simulink model "TestModel"  (R2022b)
settings: Solver=VariableStepAuto  StartTime=0.0  StopTime=10.0  RelTol=1e-3
settings Model: Creator=emanuelevitetta  LastModifiedBy=emanuelevitetta

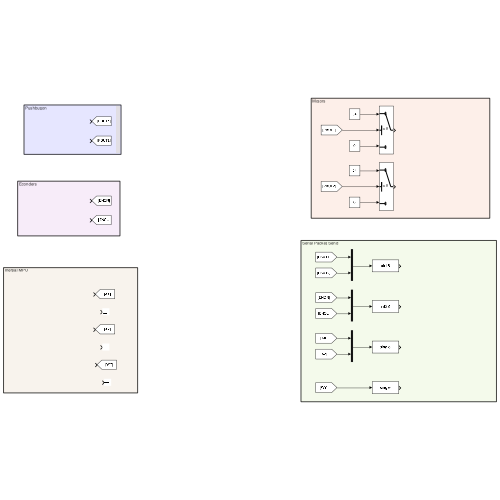
[thumbnail: Simulink's stored preview of the top-level diagram]
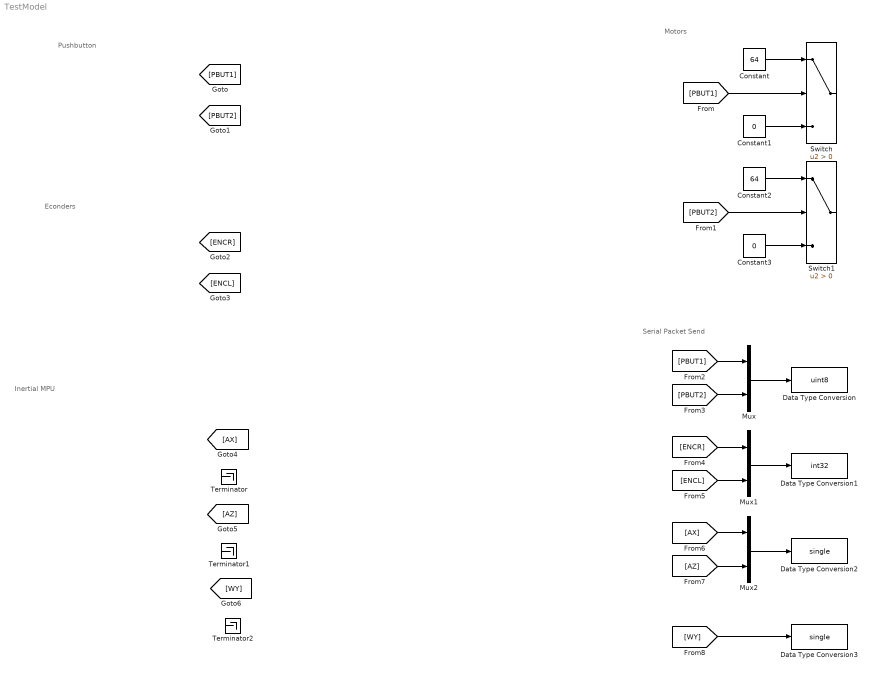
== system TestModel ==
  note: Inertial MPU
  note: Econders
  note: Serial Packet Send
  note: Motors
  note: Pushbutton
  Constant : Constant  Value=64
  Constant1 : Constant  Value=0
  Constant2 : Constant  Value=64
  Constant3 : Constant  Value=0
  Data Type Conversion : DataTypeConversion  OutDataTypeStr=uint8  SaturateOnIntegerOverflow=off  RndMeth=Floor
  Data Type Conversion1 : DataTypeConversion  OutDataTypeStr=int32  SaturateOnIntegerOverflow=off  RndMeth=Floor
  Data Type Conversion2 : DataTypeConversion  OutDataTypeStr=single  SaturateOnIntegerOverflow=off  RndMeth=Floor
  Data Type Conversion3 : DataTypeConversion  OutDataTypeStr=single  SaturateOnIntegerOverflow=off  RndMeth=Floor
  Mux : Mux  Inputs=2
  Mux1 : Mux  Inputs=2
  Mux2 : Mux  Inputs=2
  Switch : Switch  Criteria=u2 > Threshold  SaturateOnIntegerOverflow=off  InputSameDT=off
  Switch1 : Switch  Criteria=u2 > Threshold  SaturateOnIntegerOverflow=off  InputSameDT=off
  Terminator : Terminator
  Terminator1 : Terminator
  Terminator2 : Terminator
  wires:
  Constant/1 -> Switch/1
  Constant1/1 -> Switch/3
  [PBUT1] -> Switch/2
  Constant2/1 -> Switch1/1
  Constant3/1 -> Switch1/3
  [PBUT2] -> Switch1/2
  [PBUT1] -> Mux/1
  [PBUT2] -> Mux/2
  Mux/1 -> Data Type Conversion/1
  [ENCL] -> Mux1/2
  [ENCR] -> Mux1/1
  Mux1/1 -> Data Type Conversion1/1
  Mux2/1 -> Data Type Conversion2/1
  [AZ] -> Mux2/2
  [AX] -> Mux2/1
  [WY] -> Data Type Conversion3/1
